simulink model "AccSim_base"  (R2021b)
settings: Solver=ode4  StartTime=0.0  StopTime=5  FixedStep=0.0001  MaxStep=1e-3  RelTol=1e-3
values from neighbouring files (symbols this model uses):
  Brake_Factor = 0.66    [VehicleParams20_ver230707.m]
  Cd = Cd/(40/3.6)^2    (= 0.6885)    [VehicleParams20_ver230707.m]
  cPiston_Area_F = 2*pi*(0.0254/2)^2    (= 0.00101341495819)    [VehicleParams20_ver230707.m]
  cPiston_Area_R = 2*pi*(0.0254/2)^2    (= 0.00101341495819)    [VehicleParams20_ver230707.m]
  eff_Radius_F = (180/2-13.5)/1000    (= 0.0765)    [VehicleParams20_ver230707.m]
  eff_Radius_R = (180/2-13.5)/1000    (= 0.0765)    [VehicleParams20_ver230707.m]
  Fd = 60*2    (= 120)    [VehicleParams20_ver230707.m]
  g = 9.80665    [VehicleParams20_ver230707.m]
  gear_f = 13.75    [VehicleParams20_ver230707.m]
  gear_r = 13.75    [VehicleParams20_ver230707.m]
  HV_voltage = 600    [VehicleParams20_ver230707.m]
  M = 200+60    (= 260)    [VehicleParams20_ver230707.m]
  Mwf = Iwf/Rwf/Rwf    (= 3.82716814816)    [VehicleParams20_ver230707.m]
  Mwr = Iwr/Rwr/Rwr    (= 3.82716814816)    [VehicleParams20_ver230707.m]
  Rwf = 18*(25.4/1000)/2    (= 0.2286)    [VehicleParams20_ver230707.m]
  Rwr = 18*(25.4/1000)/2    (= 0.2286)    [VehicleParams20_ver230707.m]
libraries: rtican x12, simulink x4, dspstat3 x1
(part 3 of 3)

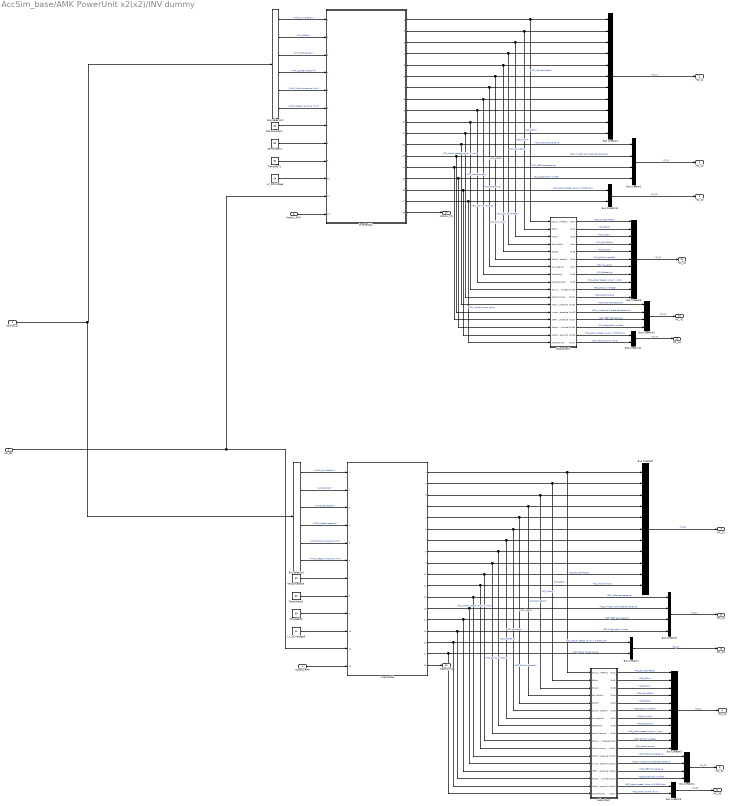
== system AccSim_base/AMK PowerUnit x2(x2)/INV dummy ==
  HV_DC : Inport
  CAN to Inv : Inport  Port=2
  Motor1_RPM : Inport  Port=3
  Motor3_RPM : Inport  Port=4
  Bus Creator{1,3,8..9} (4 alike) : BusCreator  Inputs=11
  Bus Creator{2,4,6,10} (4 alike) : BusCreator  Inputs=4
  Bus Creator{5,7,11..12} (4 alike) : BusCreator  Inputs=2
  Bus Selector1 : BusSelector  OutputSignals=AMK_21.AMK2_bInverterOn,AMK_21.AMK_bDcOn,AMK_21.AMK2_bEnableOn,AMK_21.AMK2_Speed setpoint,AMK_21.AMK2_Positive torque limit,AMK_21.AMK2_Negative torque limit
  Bus Selector3 : BusSelector  OutputSignals=AMK_11.AMK1_bInverterOn,AMK_11.AMK_bDcOn,AMK_11.AMK1_bEnableOn,AMK_11.AMK1_Speed setpoint,AMK_11.AMK1_Positive torque limit,AMK_11.AMK1_Negative torque limit
  Inverter1&4 : Subsystem  ReferencedSubsystem=PowerUnit_AMK
  Inverter2&3 : Subsystem  ReferencedSubsystem=PowerUnit_AMK
  LV_DCVoltage : Constant  Value=24
  LV_DCVoltage3 : Constant  Value=24
  Subsystem : Subsystem
  Subsystem1 : Subsystem
  TempIGBT1 : Constant  Value=30
  TempIGBT3 : Constant  Value=30
  "TempInverter1 " : Constant  Value=30
  TempInverter3 : Constant  Value=30
  TempMoter1 : Constant  Value=30
  TempMoter3 : Constant  Value=30
  MC_11 : Outport  VectorParamsAs1DForOutWhenUnconnected=off
  MC_12 : Outport  Port=2  VectorParamsAs1DForOutWhenUnconnected=off
  MC_13 : Outport  Port=3  VectorParamsAs1DForOutWhenUnconnected=off
  MC_31 : Outport  Port=4  VectorParamsAs1DForOutWhenUnconnected=off
  MC_32 : Outport  Port=5  VectorParamsAs1DForOutWhenUnconnected=off
  MC_33 : Outport  Port=6  VectorParamsAs1DForOutWhenUnconnected=off
  MC_21 : Outport  Port=7  VectorParamsAs1DForOutWhenUnconnected=off
  MC_22 : Outport  Port=8  VectorParamsAs1DForOutWhenUnconnected=off
  MC_23 : Outport  Port=9  VectorParamsAs1DForOutWhenUnconnected=off
  MC_41 : Outport  Port=10  VectorParamsAs1DForOutWhenUnconnected=off
  MC_42 : Outport  Port=11  VectorParamsAs1DForOutWhenUnconnected=off
  MC_43 : Outport  Port=12  VectorParamsAs1DForOutWhenUnconnected=off
  Motor1_Trq : Outport  Port=13  VectorParamsAs1DForOutWhenUnconnected=off
  Motor3_Trq : Outport  Port=14  VectorParamsAs1DForOutWhenUnconnected=off
  wires:
  TempMoter1/1 -> Inverter1&4/8
  TempIGBT1/1 -> Inverter1&4/9
  LV_DCVoltage/1 -> Inverter1&4/10
  "TempInverter1 "/1 -> Inverter1&4/7
  Inverter1&4/4 -> Subsystem1/4(bQuitDcOn), Bus Creator1/4  "MC1_bQuitDcOn"
  HV_DC/1 -> Inverter1&4/11, Inverter2&3/11
  Bus Selector3/6 -> Inverter1&4/6  "<AMK1_Negative torque limit>"
  CAN to Inv/1 -> Bus Selector1/1, Bus Selector3/1
  Bus Selector3/3 -> Inverter1&4/3  "<AMK1_bEnableOn>"
  Bus Selector3/5 -> Inverter1&4/5  "<AMK1_Positive torque limit>"
  Bus Selector3/1 -> Inverter1&4/1  "<AMK1_bInverterOn>"
  Bus Selector3/2 -> Inverter1&4/2  "<AMK_bDcOn>"
  Bus Selector3/4 -> Inverter1&4/4  "<AMK1_Speed setpoint>"
  TempMoter3/1 -> Inverter2&3/8
  TempIGBT3/1 -> Inverter2&3/9
  LV_DCVoltage3/1 -> Inverter2&3/10
  TempInverter3/1 -> Inverter2&3/7
  Bus Selector1/3 -> Inverter2&3/3  "<AMK2_bEnableOn>"
  Bus Selector1/1 -> Inverter2&3/1  "<AMK2_bInverterOn>"
  Bus Selector1/2 -> Inverter2&3/2  "<AMK_bDcOn>"
  Bus Selector1/4 -> Inverter2&3/4  "<AMK2_Speed setpoint>"
  Bus Selector1/5 -> Inverter2&3/5  "<AMK2_Positive torque limit>"
  Bus Selector1/6 -> Inverter2&3/6  "<AMK2_Negative torque limit>"
  Inverter2&3/18 -> Motor3_Trq/1
  Motor1_RPM/1 -> Inverter1&4/12
  Motor3_RPM/1 -> Inverter2&3/12
  Inverter1&4/18 -> Motor1_Trq/1
  Bus Creator7/1 -> MC_23/1  "MC_23"
  Bus Creator6/1 -> MC_22/1  "MC_22"
  Bus Creator8/1 -> MC_21/1  "MC_21"
  Inverter2&3/14 -> Subsystem/14(IGBT temperature), Bus Creator6/3  "MC2_IGBT temperature"
  Inverter2&3/16 -> Subsystem/16(ActualVerocity2), Bus Creator7/1  "MC2_Actual speed value in 0;0001/rpm"
  Inverter2&3/13 -> Subsystem/13(Inverter temperature), Bus Creator6/2  "MC2_Inverter cold plate temperature"
  Inverter2&3/8 -> Subsystem/8(bDerating), Bus Creator8/8  "MC2_bDerating"
  Inverter2&3/6 -> Subsystem/6(bQuitInverterOn), Bus Creator8/6  "MC2_bQuitInverterOn"
  Inverter2&3/10 -> Subsystem/10(DC bus voltage), Bus Creator8/10  "MC2_DC bus voltage"
  Inverter2&3/12 -> Subsystem/12(Motor temperature), Bus Creator6/1  "MC2_Motor temperature"
  Inverter2&3/2 -> Subsystem/2(bError), Bus Creator8/2  "MC2_bError"
  Inverter2&3/7 -> Subsystem/7(bInverterOn), Bus Creator8/7  "MC2_bInverOn"
  Inverter2&3/17 -> Bus Creator7/2, Subsystem/17(ActualPower)  "MC2_Actual power value"
  Inverter2&3/3 -> Subsystem/3(bWarn), Bus Creator8/3  "MC2_bWarn"
  Inverter2&3/1 -> Subsystem/1(bSystemReady), Bus Creator8/1  "MC2_bSystemReady"
  Inverter2&3/11 -> Subsystem/11(Actual torque), Bus Creator8/11  "MC2_Actual torque"
  Inverter2&3/15 -> Subsystem/15(Diagnostic number), Bus Creator6/4  "MC2_Diagnostic number"
  Inverter2&3/4 -> Subsystem/4(bQuitDcOn), Bus Creator8/4  "MC2_bQuitDcOn"
  Inverter2&3/5 -> Subsystem/5(bDcOn), Bus Creator8/5  "MC2_bDcOn"
  Inverter2&3/9 -> Subsystem/9(ActualVerocity), Bus Creator8/9  "MC2_Actual speed value in 1/rpm"
  Inverter1&4/13 -> Subsystem1/13(Inverter temperature), Bus Creator2/2  "MC1_Inverter cold plate temperature"
  Inverter1&4/6 -> Subsystem1/6(bQuitInverterOn), Bus Creator1/6  "MC1_bQuitInverterOn"
  Inverter1&4/7 -> Subsystem1/7(bInverterOn), Bus Creator1/7  "MC1_bInverOn"
  Inverter1&4/15 -> Subsystem1/15(Diagnostic number), Bus Creator2/4  "MC1_Diagnostic number"
  Inverter1&4/11 -> Subsystem1/11(Actual torque), Bus Creator1/11  "MC1_Actual torque"
  Inverter1&4/3 -> Subsystem1/3(bWarn), Bus Creator1/3  "MC1_bWarn"
  Inverter1&4/2 -> Subsystem1/2(bError), Bus Creator1/2  "MC1_bError"
  Inverter1&4/12 -> Subsystem1/12(Motor temperature), Bus Creator2/1  "MC1_Motor temperature"
  Inverter1&4/8 -> Subsystem1/8(bDerating), Bus Creator1/8  "MC1_bDerating"
  Inverter1&4/17 -> Subsystem1/17(ActualPower), Bus Creator12/2  "MC1_Actual power value"
  Inverter1&4/1 -> Subsystem1/1(bSystemReady), Bus Creator1/1  "MC1_bSystemReady"
  Inverter1&4/10 -> Subsystem1/10(DC bus voltage), Bus Creator1/10  "MC1_DC bus voltage"
  Inverter1&4/14 -> Subsystem1/14(IGBT temperature), Bus Creator2/3  "MC1_IGBT temperature"
  Inverter1&4/16 -> Subsystem1/16(ActualVerocity2), Bus Creator12/1  "MC1_Actual speed value in 0;0001/rpm"
  Bus Creator12/1 -> MC_13/1  "MC_13"
  Bus Creator2/1 -> MC_12/1  "MC_12"
  Bus Creator1/1 -> MC_11/1  "MC_11"
  Inverter1&4/5 -> Subsystem1/5(bDcOn), Bus Creator1/5  "MC1_bDcOn"
  Inverter1&4/9 -> Subsystem1/9(ActualVerocity), Bus Creator1/9  "MC1_Actual speed value in 1/rpm"
  Subsystem/15(Out15) -> Bus Creator4/4  "MC3_Diagnostic number"
  Subsystem/13(Out13) -> Bus Creator4/2  "MC3_Inverter cold plate temperature"
  Subsystem/2(Out2) -> Bus Creator3/2  "MC3_bError"
  Subsystem/9(Out9) -> Bus Creator3/9  "MC3_Actual speed value in 1/rpm"
  Subsystem/7(Out7) -> Bus Creator3/7  "MC3_bInverOn"
  Subsystem/4(Out4) -> Bus Creator3/4  "MC3_bQuitDcOn"
  Subsystem/8(Out8) -> Bus Creator3/8  "MC3_bDerating"
  Subsystem/3(Out3) -> Bus Creator3/3  "MC3_bWarn"
  Subsystem/17(Out17) -> Bus Creator5/2  "MC3_Actual power value"
  Bus Creator5/1 -> MC_33/1  "MC_33"
  Subsystem/14(Out14) -> Bus Creator4/3  "MC3_IGBT temperature"
  Bus Creator4/1 -> MC_32/1  "MC_32"
  Subsystem/5(Out5) -> Bus Creator3/5  "MC3_bDcOn"
  Subsystem/12(Out12) -> Bus Creator4/1  "MC3_Motor temperature"
  Subsystem/16(Out16) -> Bus Creator5/1  "MC3_Actual speed value in 0;0001/rpm"
  Subsystem/11(Out11) -> Bus Creator3/11  "MC3_Actual torque"
  Subsystem/6(Out6) -> Bus Creator3/6  "MC3_bQuitInverterOn"
  Bus Creator3/1 -> MC_31/1  "MC_31"
  Subsystem/1(Out1) -> Bus Creator3/1  "MC3_bSystemReady"
  Subsystem/10(Out10) -> Bus Creator3/10  "MC3_DC bus voltage"
  Bus Creator11/1 -> MC_43/1  "MC_43"
  Subsystem1/7(Out7) -> Bus Creator9/7  "MC4_bInverOn"
  Subsystem1/16(Out16) -> Bus Creator11/1  "MC4_Actual speed value in 0;0001/rpm"
  Subsystem1/12(Out12) -> Bus Creator10/1  "MC4_Motor temperature"
  Subsystem1/9(Out9) -> Bus Creator9/9  "MC4_Actual speed value in 1/rpm"
  Subsystem1/5(Out5) -> Bus Creator9/5  "MC4_bDcOn"
  Subsystem1/8(Out8) -> Bus Creator9/8  "MC4_bDerating"
  Bus Creator9/1 -> MC_41/1  "MC_41"
  Subsystem1/3(Out3) -> Bus Creator9/3  "MC4_bWarn"
  Subsystem1/4(Out4) -> Bus Creator9/4  "MC4_bQuitDcOn"
  Subsystem1/14(Out14) -> Bus Creator10/3  "MC4_IGBT temperature"
  Subsystem1/1(Out1) -> Bus Creator9/1  "MC4_bSystemReady"
  Subsystem1/15(Out15) -> Bus Creator10/4  "MC4_Diagnostic number"
  Subsystem1/6(Out6) -> Bus Creator9/6  "MC4_bQuitInverterOn"
  Subsystem1/11(Out11) -> Bus Creator9/11  "MC4_Actual torque"
  Subsystem1/17(Out17) -> Bus Creator11/2  "MC4_Actual power value"
  Subsystem1/13(Out13) -> Bus Creator10/2  "MC4_Inverter cold plate temperature"
  Subsystem1/10(Out10) -> Bus Creator9/10  "MC4_DC bus voltage"
  Bus Creator10/1 -> MC_42/1  "MC_42"
  Subsystem1/2(Out2) -> Bus Creator9/2  "MC4_bError"

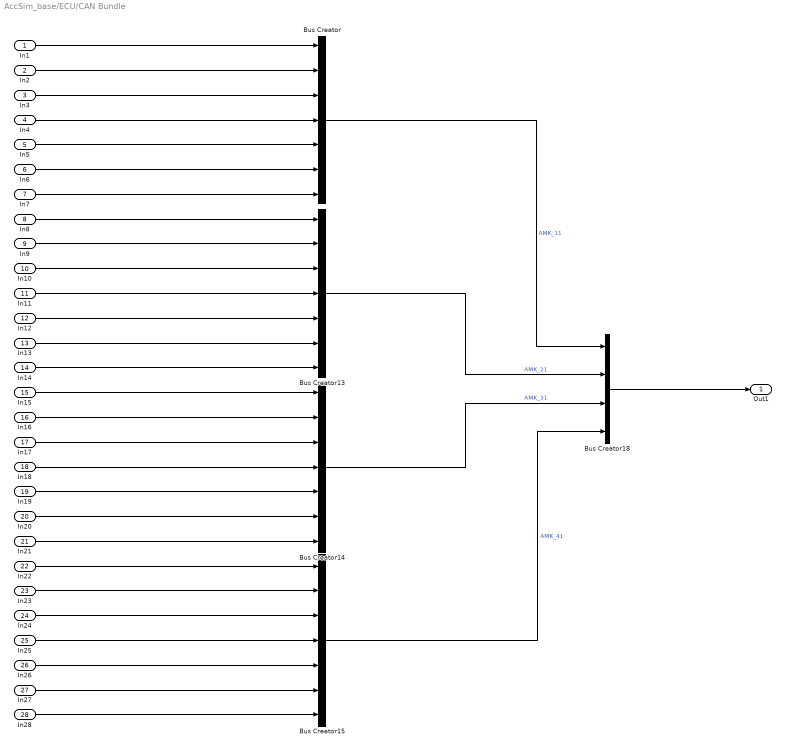
== system AccSim_base/ECU/CAN Bundle ==
  In1 : Inport
  In2 : Inport  Port=2
  In3 : Inport  Port=3
  In4 : Inport  Port=4
  In5 : Inport  Port=5
  In6 : Inport  Port=6
  In7 : Inport  Port=7
  In8 : Inport  Port=8
  In9 : Inport  Port=9
  In10 : Inport  Port=10
  In11 : Inport  Port=11
  In12 : Inport  Port=12
  In13 : Inport  Port=13
  In14 : Inport  Port=14
  In15 : Inport  Port=15
  In16 : Inport  Port=16
  In17 : Inport  Port=17
  In18 : Inport  Port=18
  In19 : Inport  Port=19
  In20 : Inport  Port=20
  In21 : Inport  Port=21
  In22 : Inport  Port=22
  In23 : Inport  Port=23
  In24 : Inport  Port=24
  In25 : Inport  Port=25
  In26 : Inport  Port=26
  In27 : Inport  Port=27
  In28 : Inport  Port=28
  Bus Creator{,13..15} (4 alike) : BusCreator  Inputs=7
  Bus Creator18 : BusCreator  Inputs=4
  Out1 : Outport  VectorParamsAs1DForOutWhenUnconnected=off
  wires:
  In7/1 -> Bus Creator/7
  In6/1 -> Bus Creator/6
  In5/1 -> Bus Creator/5
  In4/1 -> Bus Creator/4
  In3/1 -> Bus Creator/3
  In2/1 -> Bus Creator/2
  In1/1 -> Bus Creator/1
  Bus Creator18/1 -> Out1/1
  In8/1 -> Bus Creator13/1
  In18/1 -> Bus Creator14/4
  In13/1 -> Bus Creator13/6
  In28/1 -> Bus Creator15/7
  Bus Creator14/1 -> Bus Creator18/3  "AMK_31"
  In19/1 -> Bus Creator14/5
  In22/1 -> Bus Creator15/1
  In11/1 -> Bus Creator13/4
  Bus Creator/1 -> Bus Creator18/1  "AMK_11"
  In26/1 -> Bus Creator15/5
  In27/1 -> Bus Creator15/6
  In23/1 -> Bus Creator15/2
  In14/1 -> Bus Creator13/7
  In21/1 -> Bus Creator14/7
  Bus Creator15/1 -> Bus Creator18/4  "AMK_41"
  In17/1 -> Bus Creator14/3
  In25/1 -> Bus Creator15/4
  Bus Creator13/1 -> Bus Creator18/2  "AMK_21"
  In20/1 -> Bus Creator14/6
  In15/1 -> Bus Creator14/1
  In9/1 -> Bus Creator13/2
  In10/1 -> Bus Creator13/3
  In24/1 -> Bus Creator15/3
  In16/1 -> Bus Creator14/2
  In12/1 -> Bus Creator13/5

== system AccSim_base/ECU/speedlimit ==
  rpm : Inport
  kph : Inport  Port=2
  Min : MinMax  Inputs=2
  kph to motor rpm : Subsystem
  speedlimit(rpm) : Outport  VectorParamsAs1DForOutWhenUnconnected=off
  wires:
  kph to motor rpm/1(rpm) -> Min/2
  rpm/1 -> Min/1
  Min/1 -> speedlimit(rpm)/1
  kph/1 -> kph to motor rpm/1(kph)

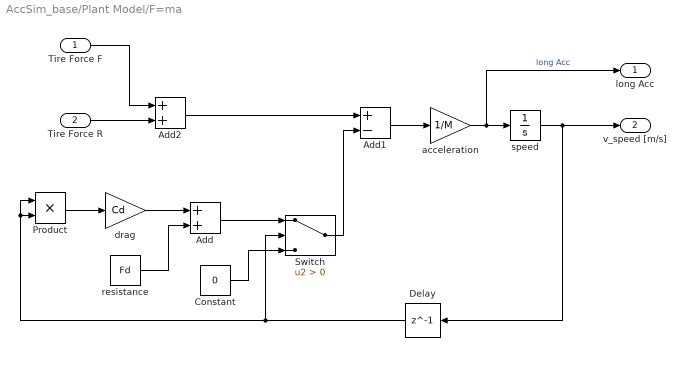
== system AccSim_base/Plant Model/F=ma ==
  Tire Force F : Inport
  Tire Force R : Inport  Port=2
  Add : Sum
  Add1 : Sum  Inputs=+-
  Add2 : Sum
  Constant : Constant  Value=0
  Delay : Delay  DelayLength=1
  Product : Product
  Switch : Switch  Criteria=u2 > Threshold
  acceleration : Gain  Gain=1/M
  drag : Gain  Gain=Cd
  resistance : Constant  Value=Fd
  speed : Integrator  LimitOutput=on  LowerSaturationLimit=0
  long Acc : Outport
  v_speed [m/s] : Outport  Port=2
  wires:
  resistance/1 -> Add/2
  Switch/1 -> Add1/2
  Constant/1 -> Switch/3
  Add1/1 -> acceleration/1
  Add2/1 -> Add1/1
  speed/1 -> v_speed [m/s]/1, Delay/1
  Add/1 -> Switch/1
  drag/1 -> Add/1
  Product/1 -> drag/1
  Tire Force R/1 -> Add2/2
  Tire Force F/1 -> Add2/1
  acceleration/1 -> long Acc/1, speed/1  "long Acc"
  Delay/1 -> Switch/2, Product/1, Product/2

== system AccSim_base/Plant Model/mu changer ==
  In1 : Inport
  In2 : Inport  Port=2
  Add4 : Sum  Inputs=+++
  Constant : Constant
  Divide : Product  Inputs=**
  Divide1 : Product  Inputs=**
  Scope1 : Scope
  Step : Step  Time=1.1  After=0.8  SampleTime=0
  Step1 : Step  After=-0.8  SampleTime=0
  Out1 : Outport
  Out2 : Outport  Port=2
  wires:
  In2/1 -> Divide1/2
  Constant/1 -> Divide1/1, Add4/1
  In1/1 -> Divide/1
  Add4/1 -> Scope1/1, Divide/2
  Step/1 -> Add4/3
  Step1/1 -> Add4/2
  Divide1/1 -> Out2/1
  Divide/1 -> Out1/1

== system AccSim_base/Sensors/NoiseGenerater1 ==
  note: SBGの説明書
      | Ellipse-N
      | Velocity Accuracy : 0.1m/s
  X : Inport
  Add : Sum  Inputs=+++
  Constant : Constant  Value=-0.1
  Gain : Gain  Gain=0
  Gain1 : Gain
  NoiseGenerater RMS0.1 : RandomNumber  Variance=0.01  SampleTime=0.001
  On/Off : Gain  Gain=0
  Scope : Scope  NumInputPorts=2
  X+X' : Outport  VectorParamsAs1DForOutWhenUnconnected=off
  wires:
  X/1 -> Gain1/1
  Add/1 -> X+X'/1  "X+X'"
  NoiseGenerater RMS0.1/1 -> Gain/1
  Gain/1 -> Add/2
  Constant/1 -> On/Off/1
  On/Off/1 -> Scope/2, Add/3
  Gain1/1 -> Scope/1, Add/1

== system AccSim_base/Sensors/NoiseGenerater2 ==
  note: SBGの説明書
      | Ellipse-N
      | Acc
      | In run bias instability : 3microg
      | 分散は適当
  X : Inport
  Add : Sum
  Gain : Gain  Gain=0
  Random Number : RandomNumber  Mean=14*10^-6  Variance=0.0001  SampleTime=0.001
  Scope : Scope  NumInputPorts=2
  X+X' : Outport  VectorParamsAs1DForOutWhenUnconnected=off
  wires:
  Random Number/1 -> Gain/1
  Add/1 -> X+X'/1, Scope/1  "X+X'"
  X/1 -> Add/1, Scope/2
  Gain/1 -> Add/2

== system AccSim_base/Sensors/NoiseGenerater3 ==
  note: SBGの説明書
      | Ellipse-N
      | Acc
      | In run bias instability : 3microg
      | 分散は適当
  X : Inport
  Add : Sum
  Gain : Gain  Gain=0
  Random Number : RandomNumber  Mean=14*10^-6*9.8  Variance=0.0001  SampleTime=0.001
  Scope : Scope  NumInputPorts=2
  X+X' : Outport  VectorParamsAs1DForOutWhenUnconnected=off
  wires:
  X/1 -> Scope/2, Add/1
  Add/1 -> Scope/1, X+X'/1  "X+X'"
  Random Number/1 -> Gain/1
  Gain/1 -> Add/2

== system AccSim_base/for Scope/80kW limit Judge ==
  Power : Inport
  Compare To Constant : simulink/Logic and Bit Operations/Compare To Constant  relop=>=  const=80000  OutDataTypeStr=boolean
  Delay : Delay  DelayLength=1
  Delay1 : Delay  DelayLength=1
  Max : MinMax  Function=max  Inputs=2
  Max1 : MinMax  Function=max  Inputs=2
  Moving Average : dspstat3/Moving Average  Method=Sliding window  ForgettingFactorPort=off  SpecifyWindowLength=on  WindowLength=100  ForgettingFactor=0.9  SimulateUsing=Code generation
  Judge : Outport  VectorParamsAs1DForOutWhenUnconnected=off
  wires:
  Moving Average/1 -> Max/1
  Max/1 -> Compare To Constant/1, Delay/1
  Power/1 -> Moving Average/1
  Delay/1 -> Max/2
  Delay1/1 -> Max1/2
  Max1/1 -> Delay1/1, Judge/1
  Compare To Constant/1 -> Max1/1

== system AccSim_base/for Scope/Acc Timer ==
  Long G : Inport
  Add : Sum  Inputs=+-
  Compare To Constant : simulink/Logic and Bit Operations/Compare To Constant  relop=<=  const=75  OutDataTypeStr=boolean
  Compare To Constant1 : simulink/Logic and Bit Operations/Compare To Constant  relop=<=  const=0.3  OutDataTypeStr=boolean
  Data Type Conversion : DataTypeConversion  OutDataTypeStr=double
  Data Type Conversion1 : DataTypeConversion  OutDataTypeStr=double
  Gain : Gain  Gain=g
  Integrator{,1..3} (4 alike) : Integrator
  fin time : Display
  fin time1 : Display
  Acc Time : Outport  VectorParamsAs1DForOutWhenUnconnected=off
  wires:
  Compare To Constant/1 -> Data Type Conversion/1
  Data Type Conversion/1 -> Integrator1/1
  Integrator1/1 -> fin time/1, Add/1
  Long G/1 -> Gain/1
  Integrator2/1 -> Integrator/1
  Gain/1 -> Integrator2/1
  Add/1 -> Acc Time/1
  Integrator3/1 -> Add/2, fin time1/1
  Compare To Constant1/1 -> Data Type Conversion1/1
  Data Type Conversion1/1 -> Integrator3/1
  Integrator/1 -> Compare To Constant1/1, Compare To Constant/1

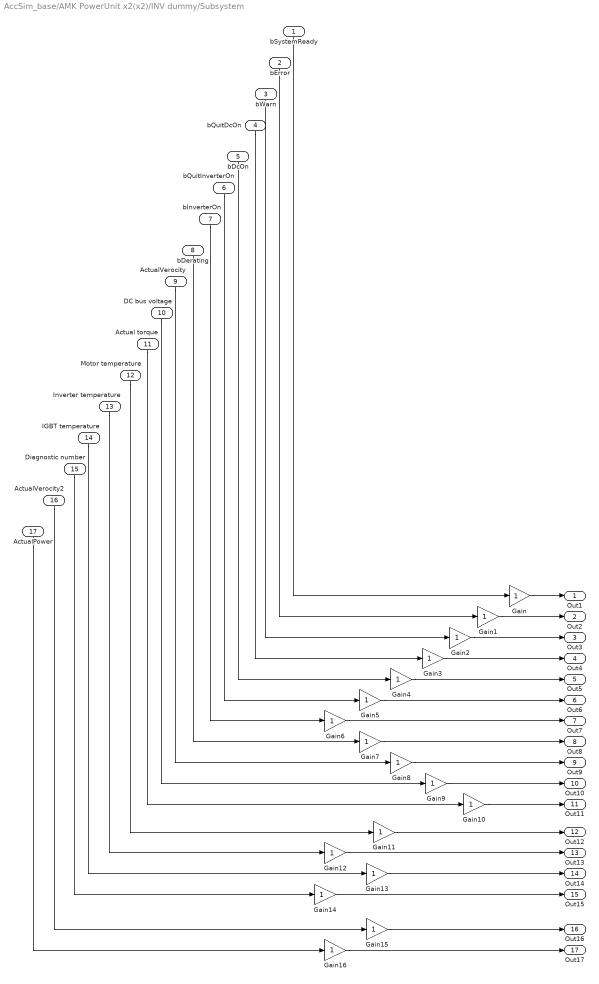
== system AccSim_base/AMK PowerUnit x2(x2)/INV dummy/Subsystem ==
  bSystemReady : Inport
  bError : Inport  Port=2
  bWarn : Inport  Port=3
  bQuitDcOn : Inport  Port=4
  bDcOn : Inport  Port=5
  bQuitInverterOn : Inport  Port=6
  bInverterOn : Inport  Port=7
  bDerating : Inport  Port=8
  ActualVerocity : Inport  Port=9
  DC bus voltage : Inport  Port=10
  Actual torque : Inport  Port=11
  Motor temperature : Inport  Port=12
  Inverter temperature : Inport  Port=13
  IGBT temperature : Inport  Port=14
  Diagnostic number : Inport  Port=15
  ActualVerocity2 : Inport  Port=16
  ActualPower : Inport  Port=17
  Gain{,1..16} (17 alike) : Gain
  Out1 : Outport  VectorParamsAs1DForOutWhenUnconnected=off
  Out2 : Outport  Port=2  VectorParamsAs1DForOutWhenUnconnected=off
  Out3 : Outport  Port=3  VectorParamsAs1DForOutWhenUnconnected=off
  Out4 : Outport  Port=4  VectorParamsAs1DForOutWhenUnconnected=off
  Out5 : Outport  Port=5  VectorParamsAs1DForOutWhenUnconnected=off
  Out6 : Outport  Port=6  VectorParamsAs1DForOutWhenUnconnected=off
  Out7 : Outport  Port=7  VectorParamsAs1DForOutWhenUnconnected=off
  Out8 : Outport  Port=8  VectorParamsAs1DForOutWhenUnconnected=off
  Out9 : Outport  Port=9  VectorParamsAs1DForOutWhenUnconnected=off
  Out10 : Outport  Port=10  VectorParamsAs1DForOutWhenUnconnected=off
  Out11 : Outport  Port=11  VectorParamsAs1DForOutWhenUnconnected=off
  Out12 : Outport  Port=12  VectorParamsAs1DForOutWhenUnconnected=off
  Out13 : Outport  Port=13  VectorParamsAs1DForOutWhenUnconnected=off
  Out14 : Outport  Port=14  VectorParamsAs1DForOutWhenUnconnected=off
  Out15 : Outport  Port=15  VectorParamsAs1DForOutWhenUnconnected=off
  Out16 : Outport  Port=16  VectorParamsAs1DForOutWhenUnconnected=off
  Out17 : Outport  Port=17  VectorParamsAs1DForOutWhenUnconnected=off
  wires:
  Gain15/1 -> Out16/1
  Inverter temperature/1 -> Gain12/1
  bDcOn/1 -> Gain4/1
  bDerating/1 -> Gain7/1
  DC bus voltage/1 -> Gain9/1
  bQuitInverterOn/1 -> Gain5/1
  bWarn/1 -> Gain2/1
  bInverterOn/1 -> Gain6/1
  Diagnostic number/1 -> Gain14/1
  ActualVerocity2/1 -> Gain15/1
  ActualPower/1 -> Gain16/1
  bError/1 -> Gain1/1
  bQuitDcOn/1 -> Gain3/1
  bSystemReady/1 -> Gain/1
  IGBT temperature/1 -> Gain13/1
  ActualVerocity/1 -> Gain8/1
  Motor temperature/1 -> Gain11/1
  Actual torque/1 -> Gain10/1
  Gain5/1 -> Out6/1
  Gain12/1 -> Out13/1
  Gain9/1 -> Out10/1
  Gain10/1 -> Out11/1
  Gain13/1 -> Out14/1
  Gain14/1 -> Out15/1
  Gain3/1 -> Out4/1
  Gain16/1 -> Out17/1
  Gain4/1 -> Out5/1
  Gain8/1 -> Out9/1
  Gain7/1 -> Out8/1
  Gain1/1 -> Out2/1
  Gain6/1 -> Out7/1
  Gain2/1 -> Out3/1
  Gain11/1 -> Out12/1
  Gain/1 -> Out1/1

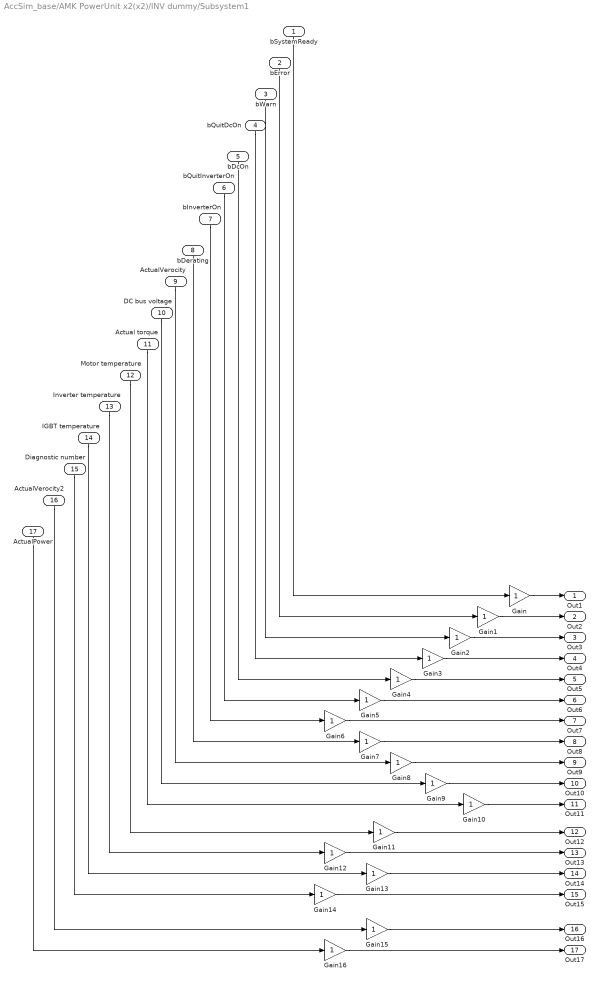
== system AccSim_base/AMK PowerUnit x2(x2)/INV dummy/Subsystem1 ==
  bSystemReady : Inport
  bError : Inport  Port=2
  bWarn : Inport  Port=3
  bQuitDcOn : Inport  Port=4
  bDcOn : Inport  Port=5
  bQuitInverterOn : Inport  Port=6
  bInverterOn : Inport  Port=7
  bDerating : Inport  Port=8
  ActualVerocity : Inport  Port=9
  DC bus voltage : Inport  Port=10
  Actual torque : Inport  Port=11
  Motor temperature : Inport  Port=12
  Inverter temperature : Inport  Port=13
  IGBT temperature : Inport  Port=14
  Diagnostic number : Inport  Port=15
  ActualVerocity2 : Inport  Port=16
  ActualPower : Inport  Port=17
  Gain{,1..16} (17 alike) : Gain
  Out1 : Outport  VectorParamsAs1DForOutWhenUnconnected=off
  Out2 : Outport  Port=2  VectorParamsAs1DForOutWhenUnconnected=off
  Out3 : Outport  Port=3  VectorParamsAs1DForOutWhenUnconnected=off
  Out4 : Outport  Port=4  VectorParamsAs1DForOutWhenUnconnected=off
  Out5 : Outport  Port=5  VectorParamsAs1DForOutWhenUnconnected=off
  Out6 : Outport  Port=6  VectorParamsAs1DForOutWhenUnconnected=off
  Out7 : Outport  Port=7  VectorParamsAs1DForOutWhenUnconnected=off
  Out8 : Outport  Port=8  VectorParamsAs1DForOutWhenUnconnected=off
  Out9 : Outport  Port=9  VectorParamsAs1DForOutWhenUnconnected=off
  Out10 : Outport  Port=10  VectorParamsAs1DForOutWhenUnconnected=off
  Out11 : Outport  Port=11  VectorParamsAs1DForOutWhenUnconnected=off
  Out12 : Outport  Port=12  VectorParamsAs1DForOutWhenUnconnected=off
  Out13 : Outport  Port=13  VectorParamsAs1DForOutWhenUnconnected=off
  Out14 : Outport  Port=14  VectorParamsAs1DForOutWhenUnconnected=off
  Out15 : Outport  Port=15  VectorParamsAs1DForOutWhenUnconnected=off
  Out16 : Outport  Port=16  VectorParamsAs1DForOutWhenUnconnected=off
  Out17 : Outport  Port=17  VectorParamsAs1DForOutWhenUnconnected=off
  wires:
  Gain15/1 -> Out16/1
  Inverter temperature/1 -> Gain12/1
  bDcOn/1 -> Gain4/1
  bDerating/1 -> Gain7/1
  DC bus voltage/1 -> Gain9/1
  bQuitInverterOn/1 -> Gain5/1
  bWarn/1 -> Gain2/1
  bInverterOn/1 -> Gain6/1
  Diagnostic number/1 -> Gain14/1
  ActualVerocity2/1 -> Gain15/1
  ActualPower/1 -> Gain16/1
  bError/1 -> Gain1/1
  bQuitDcOn/1 -> Gain3/1
  bSystemReady/1 -> Gain/1
  IGBT temperature/1 -> Gain13/1
  ActualVerocity/1 -> Gain8/1
  Motor temperature/1 -> Gain11/1
  Actual torque/1 -> Gain10/1
  Gain5/1 -> Out6/1
  Gain12/1 -> Out13/1
  Gain9/1 -> Out10/1
  Gain10/1 -> Out11/1
  Gain13/1 -> Out14/1
  Gain14/1 -> Out15/1
  Gain3/1 -> Out4/1
  Gain16/1 -> Out17/1
  Gain4/1 -> Out5/1
  Gain8/1 -> Out9/1
  Gain7/1 -> Out8/1
  Gain1/1 -> Out2/1
  Gain6/1 -> Out7/1
  Gain2/1 -> Out3/1
  Gain11/1 -> Out12/1
  Gain/1 -> Out1/1

== system AccSim_base/ECU/speedlimit/kph to motor rpm ==
  kph : Inport
  Gear : Gain  Gain=13.75
  to m/s : Gain  Gain=1000/3600
  toTire_rpm : Gain  Gain=60/(2*pi*0.228)
  rpm : Outport  VectorParamsAs1DForOutWhenUnconnected=off
  wires:
  Gear/1 -> rpm/1
  to m/s/1 -> toTire_rpm/1
  toTire_rpm/1 -> Gear/1
  kph/1 -> to m/s/1
